simulink model "System_Composer_Sequence_Diagram_Example"  (R2025b)
settings: Solver=VariableStepAuto  StartTime=0.0  StopTime=10.0  RelTol=1e-3
model workspace (MAT data in the model file):
  ValueType = Simulink.ValueType
settings Model: Creator=georg  LastModifiedBy=P28500

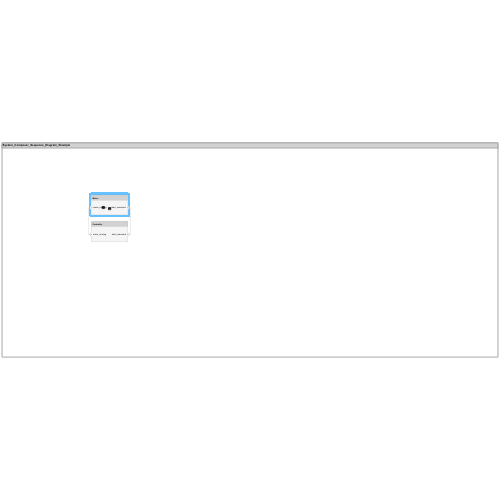
[thumbnail: Simulink's stored preview of the top-level diagram]
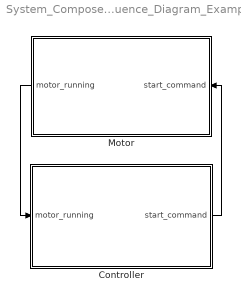
== system System_Composer_Sequence_Diagram_Example ==
  Controller : Subsystem
      settings: PortSchema="{\"entries\":[{\"content\":{\"headerSize\":26,\"margin\":15,\"minimumSpacing\":25,\"sides\":[{\"content\":{\"connectorIds\":[\"In1\"]},\"type\":\"ConnectorPlacement.EquallySpacedRectSide\",\"uuid\":\"f2b8d0f2-7f5d-455f-be3b-bebc8923d0ca\"},{\"content\":{\"connectorIds\":[\"Out1\"],\"side\":\"RIGHT\"},\"type\":\"ConnectorPlacement.EquallySpacedRectSide\",\"uuid\":\"31a0e29f-9864-4338-a782-8b947d3fedba\"},{\"content\":{\"side\":\"TOP\"},\"type\":\"ConnectorPlacement.EquallySpacedRectSide\",\"uuid\":\"4942ece6-1afd-4d8c-8cd3-26dd6f5f24c0\"},{\"content\":{\"side\":\"BOTTOM\"},\"type\":\"ConnectorPlacement.EquallySpacedRectSide\",\"uuid\":\"80afb963-df9b-44b8-a0ac-6ec440b7f0e9\"}]},\"type\":\"ConnectorPlacement.EquallySpacedConnector\",\"uuid\":\"76591b92-e423-4447-934b-80faf59083dd\"}],\"packageUris\":[\"http://schema.mathworks.com/mf0/Connector/R2020b\"],\"version\":\"1.0\"}"
  Motor : Subsystem
      settings: PortSchema="{\"entries\":[{\"content\":{\"headerSize\":26,\"margin\":15,\"minimumSpacing\":25,\"sides\":[{\"content\":{\"connectorIds\":[\"Out1\"]},\"type\":\"ConnectorPlacement.EquallySpacedRectSide\",\"uuid\":\"f2b8d0f2-7f5d-455f-be3b-bebc8923d0ca\"},{\"content\":{\"connectorIds\":[\"In1\"],\"side\":\"RIGHT\"},\"type\":\"ConnectorPlacement.EquallySpacedRectSide\",\"uuid\":\"31a0e29f-9864-4338-a782-8b947d3fedba\"},{\"content\":{\"side\":\"TOP\"},\"type\":\"ConnectorPlacement.EquallySpacedRectSide\",\"uuid\":\"4942ece6-1afd-4d8c-8cd3-26dd6f5f24c0\"},{\"content\":{\"side\":\"BOTTOM\"},\"type\":\"ConnectorPlacement.EquallySpacedRectSide\",\"uuid\":\"11339b56-b980-4906-a7d5-ffb99b837df0\"}]},\"type\":\"ConnectorPlacement.EquallySpacedConnector\",\"uuid\":\"76591b92-e423-4447-934b-80faf59083dd\"}],\"packageUris\":[\"http://schema.mathworks.com/mf0/Connector/R2020b\"],\"version\":\"1.0\"}"
  wires:
  Motor/1(motor_running) -> Controller/1(motor_running)
  Controller/1(start_command) -> Motor/1(start_command)

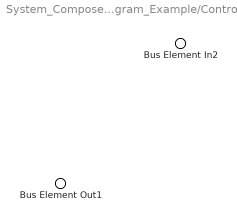
== system System_Composer_Sequence_Diagram_Example/Controller ==
  Bus Element In2 : Inport  PortName=motor_running
  Bus Element Out1 : Outport  PortName=start_command

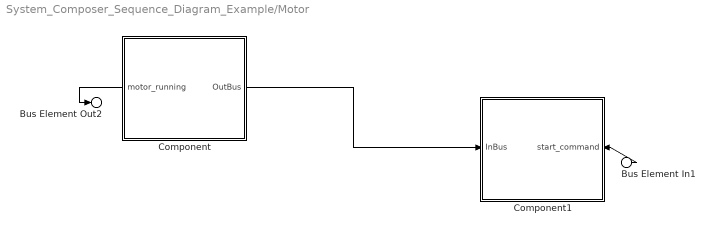
== system System_Composer_Sequence_Diagram_Example/Motor ==
  Bus Element In1 : Inport  PortName=start_command
  Component : Stateflow chart  TreatAsAtomicUnit=on
      settings: PortSchema="{\"entries\":[{\"content\":{\"headerSize\":26,\"margin\":15,\"minimumSpacing\":25,\"sides\":[{\"content\":{\"connectorIds\":[\"Out1\"]},\"type\":\"ConnectorPlacement.EquallySpacedRectSide\",\"uuid\":\"77e644ac-cc1e-4164-b9e3-38dad8eef4d2\"},{\"content\":{\"connectorIds\":[\"Out2\"],\"side\":\"RIGHT\"},\"type\":\"ConnectorPlacement.EquallySpacedRectSide\",\"uuid\":\"2140499f-a52a-4e87-b71c-4412cc790c2d\"},{\"content\":{\"side\":\"TOP\"},\"type\":\"ConnectorPlacement.EquallySpacedRectSide\",\"uuid\":\"76ef3de7-908f-42ac-9497-7966aee48685\"}]},\"type\":\"ConnectorPlacement.EquallySpacedConnector\",\"uuid\":\"37f7d6e2-2535-4b8f-a441-6386f47bce9d\"}],\"packageUris\":[\"http://schema.mathworks.com/mf0/Connector/R2020b\"],\"version\":\"1.0\"}"
  Component1 : Stateflow chart  TreatAsAtomicUnit=on
      settings: PortSchema="{\"entries\":[{\"content\":{\"headerSize\":26,\"margin\":15,\"minimumSpacing\":25,\"sides\":[{\"content\":{\"connectorIds\":[\"In1\"]},\"type\":\"ConnectorPlacement.EquallySpacedRectSide\",\"uuid\":\"77e644ac-cc1e-4164-b9e3-38dad8eef4d2\"},{\"content\":{\"connectorIds\":[\"In2\"],\"side\":\"RIGHT\"},\"type\":\"ConnectorPlacement.EquallySpacedRectSide\",\"uuid\":\"2140499f-a52a-4e87-b71c-4412cc790c2d\"},{\"content\":{\"side\":\"TOP\"},\"type\":\"ConnectorPlacement.EquallySpacedRectSide\",\"uuid\":\"76ef3de7-908f-42ac-9497-7966aee48685\"}]},\"type\":\"ConnectorPlacement.EquallySpacedConnector\",\"uuid\":\"37f7d6e2-2535-4b8f-a441-6386f47bce9d\"}],\"packageUris\":[\"http://schema.mathworks.com/mf0/Connector/R2020b\"],\"version\":\"1.0\"}"
  Bus Element Out2 : Outport  PortName=motor_running
  wires:
  Component/1(motor_running) -> Bus Element Out2/1
  Component/2(OutBus) -> Component1/1(InBus)
  Bus Element In1/1 -> Component1/2(start_command)

== stateflow chart System_Composer_Sequence_Diagram_Example/Motor/Component1 ==
  data: InBus input; start_command input

== stateflow chart System_Composer_Sequence_Diagram_Example/Motor/Component ==
  data: motor_running output; OutBus output
